simulink model "Luenberger"  (R2020a)
settings: Solver=VariableStepAuto  StartTime=0.0  StopTime=10.0  RelTol=1e-3
values from neighbouring files (symbols this model uses):
  A = [0, 1; 4.1*10^4, 0]    [Initialize_params.m]    (also in Luenberger_params.m)
  B = [0; -9.12]    [Initialize_params.m]    (also in Luenberger_params.m)
  C = [1 0;0 1]    [Initialize_params.m]    (also in Luenberger_params.m)
  L = place(A',C', eig_Kc)    [Luenberger_params.m]
undefined symbols (not defined in the file or in its folder): Kc
settings Model: Creator=prans  LastModifiedBy=prans

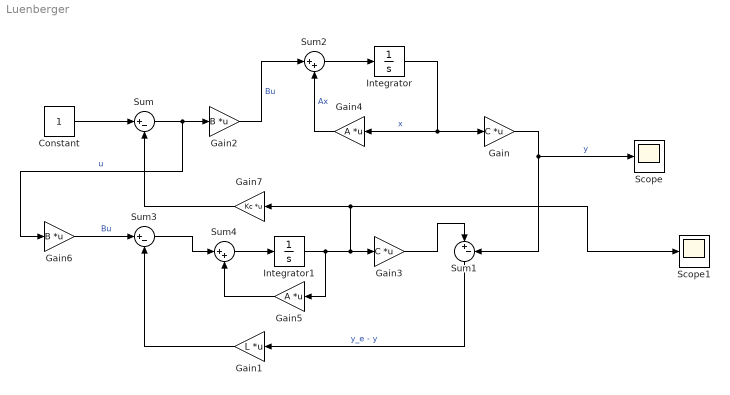
== system Luenberger ==
  Constant : Constant
  Gain : Gain  Gain=C  Multiplication=Matrix(K*u)
  Gain1 : Gain  Gain=L  Multiplication=Matrix(K*u)
  Gain2 : Gain  Gain=B  Multiplication=Matrix(K*u)
  Gain3 : Gain  Gain=C  Multiplication=Matrix(K*u)
  Gain4 : Gain  Gain=A  Multiplication=Matrix(K*u)
  Gain5 : Gain  Gain=A  Multiplication=Matrix(K*u)
  Gain6 : Gain  Gain=B  Multiplication=Matrix(K*u)
  Gain7 : Gain  Gain=Kc  Multiplication=Matrix(K*u)
  Integrator : Integrator
  Integrator1 : Integrator
  Scope : Scope
  Scope1 : Scope
  Sum : Sum  Inputs=|+-
  Sum1 : Sum  Inputs=|+-
  Sum2 : Sum  Inputs=|++
  Sum3 : Sum  Inputs=|+-
  Sum4 : Sum  Inputs=|++
  wires:
  Constant/1 -> Sum/1
  Sum/1 -> Gain2/1, Gain6/1  "u"
  Integrator/1 -> Gain4/1, Gain/1  "x"
  Gain/1 -> Sum1/2, Scope/1  "y"
  Sum1/1 -> Gain1/1  "y_e - y"
  Gain1/1 -> Sum3/2
  Sum3/1 -> Sum4/1
  Integrator1/1 -> Gain5/1, Gain7/1, Scope1/1, Gain3/1
  Gain3/1 -> Sum1/1
  Gain2/1 -> Sum2/1  "Bu"
  Sum2/1 -> Integrator/1
  Gain4/1 -> Sum2/2  "Ax"
  Gain5/1 -> Sum4/2
  Sum4/1 -> Integrator1/1
  Gain6/1 -> Sum3/1  "Bu"
  Gain7/1 -> Sum/2
